simulink model "simlink"  (R2021a)
settings: Solver=VariableStepAuto  StartTime=0.0  StopTime=500  RelTol=1e-3
settings Model: Creator=l_w_h  LastModifiedBy=l_w_h

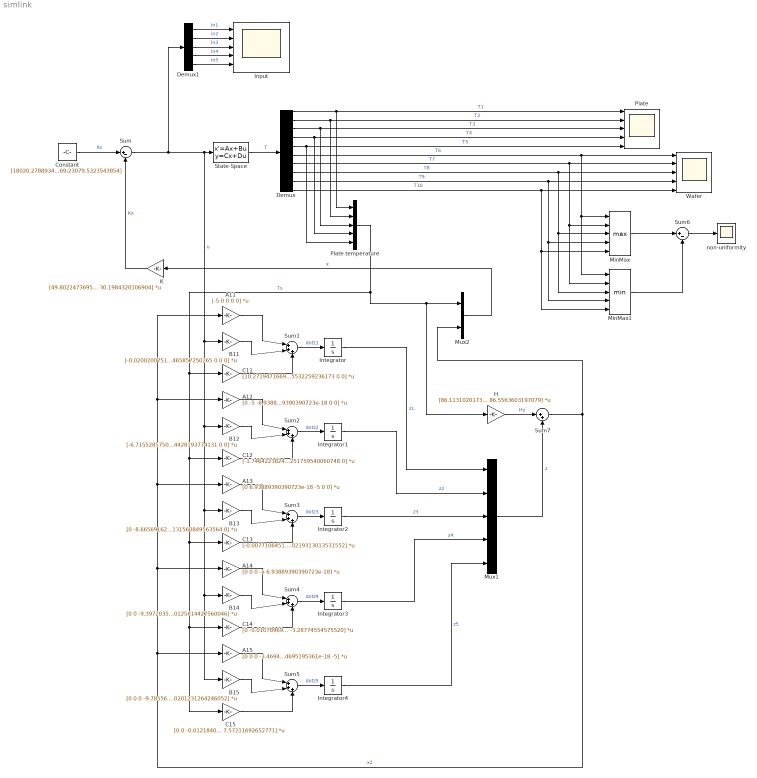
== system simlink ==
  A11 : Gain  Gain=[-5 0 0 0 0]  Multiplication=Matrix(K*u)
  A12 : Gain  Gain=[0 -5 -6.93889390390723e-18 0 0]  Multiplication=Matrix(K*u)
  A13 : Gain  Gain=[0 6.93889390390723e-18 -5 0 0]  Multiplication=Matrix(K*u)
  A14 : Gain  Gain=[0 0 0 -5 6.93889390390723e-18]  Multiplication=Matrix(K*u)
  A15 : Gain  Gain=[0 0 0 -3.46944695195361e-18 -5]  Multiplication=Matrix(K*u)
  B11 : Gain  Gain=[-0.0200200751546151 -0.000201465857250265 0 0 0]  Multiplication=Matrix(K*u)
  B12 : Gain  Gain=[-6.71552857500885e-05 -0.0200099575323411 -0.000144428193774131 0 0]  Multiplication=Matrix(K*u)
  B13 : Gain  Gain=[0 -8.66569162644783e-05 -0.0200033232460373 -0.000131560849563564 0]  Multiplication=Matrix(K*u)
  B14 : Gain  Gain=[0 0 -9.39720354025459e-05 -0.0200017545489028 -0.000125814427560046]  Multiplication=Matrix(K*u)
  B15 : Gain  Gain=[0 0 0 -9.78556658800356e-05 -0.0201231264246052]  Multiplication=Matrix(K*u)
  C11 : Gain  Gain=[10.2719471669544 -5.23926714731687 -0.0385532259236173 0 0]  Multiplication=Matrix(K*u)
  C12 : Gain  Gain=[-1.74642238243896 10.5184803661585 -3.75275523599952 -0.0251759540060748 0]  Multiplication=Matrix(K*u)
  C13 : Gain  Gain=[-0.00771064518472346 -2.25165314159971 10.6924081102485 -3.41698622839697 -0.0219313013531552]  Multiplication=Matrix(K*u)
  C14 : Gain  Gain=[0 -0.0107896945740321 -2.44070444885498 10.7334217169851 -3.28774554575520]  Multiplication=Matrix(K*u)
  C15 : Gain  Gain=[0 0 -0.0121840563073084 -2.55710591670366 7.57211692652771]  Multiplication=Matrix(K*u)
  Constant : Constant  Value=[18020.2788934933;24723.3786459106;23421.7110229547;22252.5693199369;23079.5323543854]
  Demux : Demux  Outputs=10
  Demux1 : Demux  Outputs=5
  H : Gain  Gain=[86.1131020173717 0.866572666906799 0 0 0;0.288857555635600 86.0695827082621 0.621234420380753 0 0;0 0.372740652228452 86.0410464031343 0.565887628915702 0;0 0 0.404205449225502 86.0342989071664 0.541170327886501;0 0 0 0.420910255022834 86.5563603197079]  Multiplication=Matrix(K*u)
  Input : Scope  NumInputPorts=5
  Integrator{,1..4} (5 alike) : Integrator
  K : Gain  Gain=[49.8022473695038 33.5235781775945 13.2247173971992 4.06509893620486 1.06329333966196 26.1068862875678 14.7548313801068 5.18599915321573 1.49447301664613 0.361957976085072;33.5235781775946 63.1493851548521 32.6322352469155 13.4623572093038 5.69022629558128 15.4041427758203 24.7823108653512 12.7712946613817 5.08284816231291 2.06845313919729;13.2247173971994 32.6322352469155 51.9981704332586 27.7305431966690 16.2160086562825 5.44730467849502 13.0441370972624 19.7442303110025 10.8261281656247 6.13733545717582;4.06509893620492 13.4623572093038 27.7305431966690 51.5770932284654 37.8692679195816 1.55614759006227 5.24598707214355 10.9758726966702 19.5474504815354 14.7761867507680;1.06329333966173 5.69022629558115 16.2160086562825 37.8692679195817 78.4034903515259 0.370427877347196 2.14885704726765 6.26509913513960 14.9029493646270 30.1984320106904]  Multiplication=Matrix(K*u)
  MinMax : MinMax  Function=max  Inputs=5
  MinMax1 : MinMax  Inputs=5
  Mux1 : Mux  Inputs=5
  Mux2 : Mux  Inputs=2
  Plate : Scope  NumInputPorts=5
  Plate temperature : Mux  Inputs=5
  State-Space : StateSpace  A=[-0.117855659679215 0.0620590628252506 0 0 0 0.0557965968539647 0 0 0 0;0.0206863542750835 -0.120972267946796 0.0444893168177479 0 0 0 0.0557965968539647 0 0 0;0 0.0266935900906488 -0.123015877698588 0.0405256907539742 0 0 0 0.0557965968539647 0 0;0 0 0.0289469219671245 -0.123499095427663 0.0387555766065743 0 0 0 0.0557965968539647 0;0 0 0 0.0301432262495578 -0.0860418872487965 0 0 0 0 0.0557965968539647;0.140956950866225 0 0 0 0 -0.195181962892381 0.0483518057400637 0 0 0;0 0.140956950866225 0 0 0 0.0161172685800212 -0.197610192238130 0.0346627665057913 0 0;0 0 0.140956950866225 0 0 0 0.0207976599034748 -0.199202420951047 0.0315746038952554 0;0 0 0 0.140956950866225 0 0 0 0.0225532884966110 -0.199578908263339 0.0301954626144110;0 0 0 0 0.140956950866225 0 0 0 0.0234853598112085 -0.170449658094751]  B=[0.000232485820224853 0 0 0 0;0 0.000232485820224853 0 0 0;0 0 0.000232485820224853 0 0;0 0 0 0.000232485820224853 0;0 0 0 0 0.000232485820224853;0 0 0 0 0;0 0 0 0 0;0 0 0 0 0;0 0 0 0 0;0 0 0 0 0]  C=[1 0 0 0 0 0 0 0 0 0;0 1 0 0 0 0 0 0 0 0;0 0 1 0 0 0 0 0 0 0;0 0 0 1 0 0 0 0 0 0;0 0 0 0 1 0 0 0 0 0;0 0 0 0 0 1 0 0 0 0;0 0 0 0 0 0 1 0 0 0;0 0 0 0 0 0 0 1 0 0;0 0 0 0 0 0 0 0 1 0;0 0 0 0 0 0 0 0 0 1]  D=[0 0 0 0 0;0 0 0 0 0;0 0 0 0 0;0 0 0 0 0;0 0 0 0 0;0 0 0 0 0;0 0 0 0 0;0 0 0 0 0;0 0 0 0 0;0 0 0 0 0]  InitialCondition=[114.583333333333;114.583333333333;114.583333333333;114.583333333333;114.688014403292;25;25;25;25;25]  ParameterTunability=Unconstrained
  Sum : Sum  Inputs=|+-
  Sum{1..5} (5 alike) : Sum  Inputs=|+++
  Sum6 : Sum  Inputs=|+-
  Sum7 : Sum  Inputs=|++
  Wafer : Scope  NumInputPorts=5
  non-uniformity : Scope
  wires:
  Demux/5 -> Plate temperature/5, Plate/5  "T5"
  Demux/9 -> Wafer/4, MinMax1/4, MinMax/4  "T9"
  Demux/3 -> Plate temperature/3, Plate/3  "T3"
  Demux/7 -> Wafer/2, MinMax1/2, MinMax/2  "T7"
  Demux/8 -> Wafer/3, MinMax1/3, MinMax/3  "T8"
  Demux/1 -> Plate temperature/1, Plate/1  "T1"
  Demux/2 -> Plate temperature/2, Plate/2  "T2"
  Demux/4 -> Plate temperature/4, Plate/4  "T4"
  Sum/1 -> Demux1/1, B15/1, B14/1, B13/1, B12/1, B11/1, State-Space/1  "u"
  Constant/1 -> Sum/1  "Rs"
  Plate temperature/1 -> Mux2/1, H/1, C15/1, C14/1, C13/1, C12/1, C11/1  "Ts"
  A11/1 -> Sum1/1
  B11/1 -> Sum1/2
  C11/1 -> Sum1/3
  Sum1/1 -> Integrator/1  "dotz1"
  B12/1 -> Sum2/2
  Sum2/1 -> Integrator1/1  "dotz2"
  A12/1 -> Sum2/1
  C12/1 -> Sum2/3
  Sum3/1 -> Integrator2/1  "dotz3"
  B13/1 -> Sum3/2
  A13/1 -> Sum3/1
  C13/1 -> Sum3/3
  C14/1 -> Sum4/3
  B14/1 -> Sum4/2
  A14/1 -> Sum4/1
  Sum4/1 -> Integrator3/1  "dotz4"
  A15/1 -> Sum5/1
  Sum5/1 -> Integrator4/1  "dotz5"
  B15/1 -> Sum5/2
  C15/1 -> Sum5/3
  Integrator/1 -> Mux1/1  "z1"
  Integrator1/1 -> Mux1/2  "z2"
  Integrator2/1 -> Mux1/3  "z3"
  Integrator3/1 -> Mux1/4  "z4"
  Integrator4/1 -> Mux1/5  "z5"
  K/1 -> Sum/2  "Kx"
  Mux2/1 -> K/1  "x"
  State-Space/1 -> Demux/1  "T"
  Demux/10 -> Wafer/5, MinMax1/5, MinMax/5  "T10"
  Demux/6 -> MinMax1/1, MinMax/1, Wafer/1  "T6"
  MinMax/1 -> Sum6/1
  MinMax1/1 -> Sum6/2
  Sum6/1 -> non-uniformity/1
  Demux1/1 -> Input/1  "in1"
  Demux1/2 -> Input/2  "in2"
  Demux1/3 -> Input/3  "in3"
  Demux1/4 -> Input/4  "in4"
  Demux1/5 -> Input/5  "in5"
  H/1 -> Sum7/1  "Hy"
  Mux1/1 -> Sum7/2  "z"
  Sum7/1 -> A11/1, A12/1, A13/1, A14/1, A15/1, Mux2/2  "x2"
